simulink model "HuskyFullSim_TorqueControl"  (R2025a)
settings: Solver=VariableStepAuto  StartTime=0.0  StopTime=1  RelTol=1e-5  AbsTol=1e-5  EnableMultiTasking=on
undefined symbols (not defined in the file): X, Y, Z
libraries: sm_lib x83, nesl_utility x81
(part 1 of 4)
settings Model: Creator=Prath  LastModifiedBy=Prath
settings SolverCC: AutoScaleAbsTol=off  AlgebraicLoopSolver=TrustRegion  MaxZcPerStep=1.0
settings DataIOCC: LimitDataPoints=on  MaxDataPoints=10000
settings OptimizationCC: ReuseModelBlockBuffer=off  LifeSpan=inf
settings DebuggingCC: UnconnectedInputMsg=warning  UnconnectedOutputMsg=warning  UnconnectedLineMsg=warning  AllowSymbolicDim=off  SubsystemReferenceDiagnosticForUnitTest=warning  SFUnexpectedBacktrackingDiag=warning  SFNoUnconditionalDefaultTransitionDiag=warning  SFExecutionAtInitializationDiag=none  ArithmeticOperatorsInVariantConditions=warning
settings ModelReferenceCC: EnableRefExpFcnMdlSchedulingChecks=on
settings SFSimCC: SimUseLocalCustomCode=off  CustomCodeUndefinedFunction=UseInterfaceOnly
settings RTWCC: RTWUseLocalCustomCode=off  GPUComputeCapability=3.5  DLArmComputeVersion=19.05
settings CodeAppCC: StateflowObjectComments=on
settings GRTTargetCC: TargetLangStandard=C89/C90 (ANSI)
settings ConfigComp: CovMetricSettings=dw  CovSaveCumulativeToWorkspaceVar=on  CovSaveSingleToWorkspaceVar=on  CovExternalEMLEnable=off  CovSFcnEnable=off
settings SimscapeCC: SimscapeLogType=all  SimscapeLogSimulationStatistics=on  SimscapeLogDataHistory=10000.0
settings ExplorerConfigSet: InternalSimMechanicsExplorerSettings="<ExplorerConfiguration><canonicalview>default</canonicalview><TilePanel><TileInfo><Tiles Columns=\"1\" Count=\"1\" Height=\"824\" Rows=\"1\" Width=\"1703\"><Row Weight=\"1\"/><Column Weight=\"1\"/><Tile Height=\"1\" Width=\"1\" X=\"0\" Y=\"0\"/></Tiles></TileInfo><SceneInfo><SceneViewer><IsThisViewStd><IsStandardView>off</IsStandardView><StandardViewName>Front</StandardViewName></IsThisViewStd><BGColor><R>1</R><G>1</G><B>1</B><A>1</A></BGColor><Camera><DoPerspective>off</DoPerspective><Position><X>-0.84082597181311081</X><Y>0.97301356742484102</Y><Z>-0.37165255861931379</Z></Position><Center><X>0.16436719658721111</X><Y>-0.14249902054546354</Y><Z>-0.28624750343827171</Z></Center><Up><X>0.59851844460548564</X><Y>0.58151391770421146</Y><Z>0.55101473209282714</Z></Up><XLim>0.64254437732877001</XLim><YLim>0.64254437732877001</YLim><ViewLimDist>0.01</ViewLimDist></Camera></SceneViewer></SceneInfo></TilePanel><MechEditorPanel><GfxPanelCameraMap/><Cameras/><VideoCreator><IncludeTiles>All</IncludeTiles><IncludeTime>on</IncludeTime><IncludeWorldFrame>off</IncludeWorldFrame><PlaybackSpeedRatio>1</PlaybackSpeedRatio><FrameRate>60</FrameRate><FrameSize>auto</FrameSize><VideoFormat>MPEG4</VideoFormat></VideoCreator></MechEditorPanel><PlaybackSettings><PlaybackSpeedFactor>1</PlaybackSpeedFactor></PlaybackSettings></ExplorerConfiguration>"

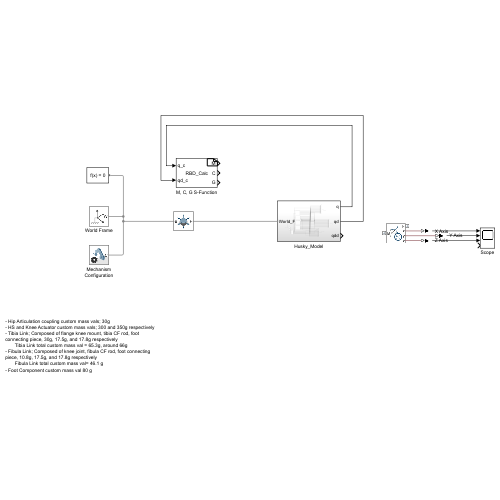
[thumbnail: Simulink's stored preview of the top-level diagram]
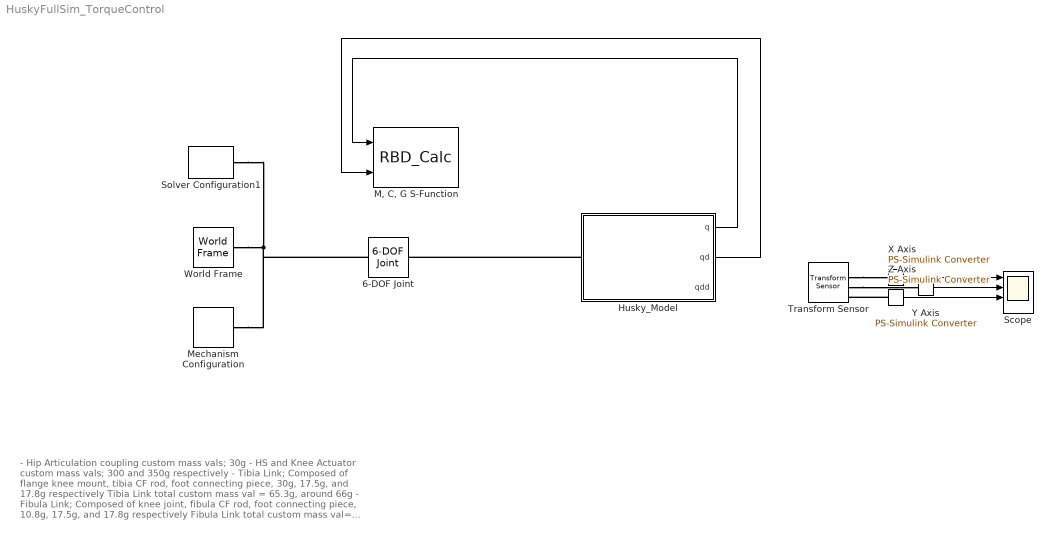
== system HuskyFullSim_TorqueControl ==
  note: - Hip Articulation coupling custom mass vals; 30g
      | - HS and Knee Actuator custom mass vals; 300 and 350g respectively
      | - Tibia Link; Composed of flange knee mount, tibia CF rod, foot connecting piece, 30g, 17.5g, and 17.8g respectively
      | Tibia Link total custom mass val = 65.3g, around 66g
      | - Fibula Link; Composed of knee joint, fibula CF rod, foot connecting piece, 10.8g, 17.5g, and 17.8g respectively
      | Fibula Link total custom mass val= 46.1 g
      | - Foot Component custom mass val 80 g
  6-DOF Joint : sm_lib/Joints/6-DOF Joint  JointMode=Normal  CompositeWrenchDir=FollowerOnBase  CompositeWrenchFrame=BaseFrame  SenseConstraintForce=off  SenseConstraintTorque=off  SenseTotalForce=off  SenseTotalTorque=off  PxPositionTargetSpecify=off  PxPositionTargetPriority=High  PxPositionTargetValue=0  PxPositionTargetValueUnits=m  PxVelocityTargetSpecify=off  PxVelocityTargetPriority=High  PxVelocityTargetValue=0  PxVelocityTargetValueUnits=m/s  PxEquilibriumPosition=0  PxEquilibriumPositionUnits=m  PxSpringStiffness=0  PxSpringStiffnessUnits=N/m  PxDampingCoefficient=0  PxDampingCoefficientUnits=N/(m/s)  PxLowerLimitSpecify=off  PxLowerLimitBound=-1  PxLowerLimitBoundUnits=m  PxLowerLimitStiffness=1e6  PxLowerLimitStiffnessUnits=N/m  PxLowerLimitDamping=1e3  PxLowerLimitDampingUnits=N/(m/s)  PxLowerLimitTransitionRegionWidth=1e-4  PxLowerLimitTransitionRegionWidthUnits=m  PxUpperLimitSpecify=off  PxUpperLimitBound=1  PxUpperLimitBoundUnits=m  PxUpperLimitStiffness=1e6  PxUpperLimitStiffnessUnits=N/m  PxUpperLimitDamping=1e3  PxUpperLimitDampingUnits=N/(m/s)  PxUpperLimitTransitionRegionWidth=1e-4  PxUpperLimitTransitionRegionWidthUnits=m  PxTorqueActuationMode=NoTorque  PxMotionActuationMode=ComputedMotion  PxSensePosition=off  PxSenseVelocity=off  PxSenseAcceleration=off  PxSenseTorqueForce=off  PxSenseLowerLimitTorqueForce=off  PxSenseUpperLimitTorqueForce=off  PyPositionTargetSpecify=off  PyPositionTargetPriority=High  PyPositionTargetValue=0  PyPositionTargetValueUnits=m  PyVelocityTargetSpecify=off  PyVelocityTargetPriority=High  PyVelocityTargetValue=0  PyVelocityTargetValueUnits=m/s  PyEquilibriumPosition=0  PyEquilibriumPositionUnits=m  PySpringStiffness=0  PySpringStiffnessUnits=N/m  PyDampingCoefficient=0  PyDampingCoefficientUnits=N/(m/s)  PyLowerLimitSpecify=off  PyLowerLimitBound=-1  PyLowerLimitBoundUnits=m  PyLowerLimitStiffness=1e6  PyLowerLimitStiffnessUnits=N/m  PyLowerLimitDamping=1e3  PyLowerLimitDampingUnits=N/(m/s)  PyLowerLimitTransitionRegionWidth=1e-4  PyLowerLimitTransitionRegionWidthUnits=m  PyUpperLimitSpecify=off  PyUpperLimitBound=1  PyUpperLimitBoundUnits=m  PyUpperLimitStiffness=1e6  PyUpperLimitStiffnessUnits=N/m  PyUpperLimitDamping=1e3  PyUpperLimitDampingUnits=N/(m/s)  PyUpperLimitTransitionRegionWidth=1e-4  PyUpperLimitTransitionRegionWidthUnits=m  PyTorqueActuationMode=NoTorque  PyMotionActuationMode=ComputedMotion  PySensePosition=off  PySenseVelocity=off  PySenseAcceleration=off  PySenseTorqueForce=off  PySenseLowerLimitTorqueForce=off  PySenseUpperLimitTorqueForce=off  PzPositionTargetSpecify=off  PzPositionTargetPriority=High  PzPositionTargetValue=0  PzPositionTargetValueUnits=m  PzVelocityTargetSpecify=off  PzVelocityTargetPriority=High  PzVelocityTargetValue=0  PzVelocityTargetValueUnits=m/s  PzEquilibriumPosition=0  PzEquilibriumPositionUnits=m  PzSpringStiffness=0  PzSpringStiffnessUnits=N/m  PzDampingCoefficient=0  PzDampingCoefficientUnits=N/(m/s)  PzLowerLimitSpecify=off  PzLowerLimitBound=-1  PzLowerLimitBoundUnits=m  PzLowerLimitStiffness=1e6  PzLowerLimitStiffnessUnits=N/m  PzLowerLimitDamping=1e3  PzLowerLimitDampingUnits=N/(m/s)  PzLowerLimitTransitionRegionWidth=1e-4  PzLowerLimitTransitionRegionWidthUnits=m  PzUpperLimitSpecify=off  PzUpperLimitBound=1  PzUpperLimitBoundUnits=m  PzUpperLimitStiffness=1e6  PzUpperLimitStiffnessUnits=N/m  PzUpperLimitDamping=1e3  PzUpperLimitDampingUnits=N/(m/s)  PzUpperLimitTransitionRegionWidth=1e-4  PzUpperLimitTransitionRegionWidthUnits=m  PzTorqueActuationMode=NoTorque  PzMotionActuationMode=ComputedMotion  PzSensePosition=off  PzSenseVelocity=off  PzSenseAcceleration=off  PzSenseTorqueForce=off  PzSenseLowerLimitTorqueForce=off  PzSenseUpperLimitTorqueForce=off  SphPositionTargetSpecify=off  SphPositionTargetPriority=High  SphPositionTargetRotationMethod=None  SphPositionTargetFollAlignAxisA=+X  SphPositionTargetBaseAlignAxisA=+Y  SphPositionTargetFollAlignAxisB=+Y  SphPositionTargetBaseAlignAxisB=+Z  SphPositionTargetRotationStandardAxis=+Z  SphPositionTargetRotationAngle=0  SphPositionTargetRotationAngleUnits=deg  SphPositionTargetRotationArbitraryAxis=[0 0 1]  SphPositionTargetRotationSequenceAxes=FollowerAxes  SphPositionTargetRotationSequence=XYX  SphPositionTargetRotationSequenceAngles=[0 0 0]  SphPositionTargetRotationSequenceAnglesUnits=deg  SphPositionTargetRotationMatrix=[1 0 0;0 1 0;0 0 1]  SphPositionTargetQuaternion=[1 0 0 0]  SphVelocityTargetSpecify=off  SphVelocityTargetPriority=High  SphVelocityTargetValue=[0 0 0]  SphVelocityTargetValueUnits=deg/s  SphVelocityTargetInFollowerFrame=on  SphEqPosRotationMethod=None  SphEqPosFollAlignAxisA=+X  SphEqPosBaseAlignAxisA=+Y  SphEqPosFollAlignAxisB=+Y  SphEqPosBaseAlignAxisB=+Z  SphEqPosRotationStandardAxis=+Z  SphEqPosRotationAngle=0  SphEqPosRotationAngleUnits=deg  SphEqPosRotationArbitraryAxis=[0 0 1]  SphEqPosRotationSequenceAxes=FollowerAxes  SphEqPosRotationSequence=XYX  SphEqPosRotationSequenceAngles=[0 0 0]  SphEqPosRotationSequenceAnglesUnits=deg  SphEqPosRotationMatrix=[1 0 0;0 1 0;0 0 1]  SphEqPosQuaternion=[1 0 0 0]  SphSpringStiffness=0  SphSpringStiffnessUnits=N*m/deg  SphDampingCoefficient=0  SphDampingCoefficientUnits=N*m/(deg/s)  SphLowerLimitSpecify=off  SphLowerLimitBound=15  SphLowerLimitBoundUnits=deg  SphLowerLimitStiffness=1e4  SphLowerLimitStiffnessUnits=N*m/deg  SphLowerLimitDamping=10  SphLowerLimitDampingUnits=N*m/(deg/s)  SphLowerLimitTransitionRegionWidth=0.1  SphLowerLimitTransitionRegionWidthUnits=deg  SphUpperLimitSpecify=off  SphUpperLimitBound=45  SphUpperLimitBoundUnits=deg  SphUpperLimitStiffness=1e4  SphUpperLimitStiffnessUnits=N*m/deg  SphUpperLimitDamping=10  SphUpperLimitDampingUnits=N*m/(deg/s)  SphUpperLimitTransitionRegionWidth=0.1  SphUpperLimitTransitionRegionWidthUnits=deg  SphTorqueActuationMode=NoTorque  SphActuateTorqueX=off  SphActuateTorqueY=off  SphActuateTorqueZ=off  SphActuateTorque=off  SphActuationFrame=BaseFrame  SphSensePosition=off  SphSenseVelocityX=off  SphSenseVelocityY=off  SphSenseVelocityZ=off  SphSenseVelocity=off  SphSenseAccelerationX=off  SphSenseAccelerationY=off  SphSenseAccelerationZ=off  SphSenseAcceleration=off  SphSenseLowerLimitTorqueMag=off  SphSenseUpperLimitTorqueMag=off  SphSensingFrame=BaseFrame
  Husky_Model : Subsystem
  "M, C, G S-Function" : S-Function  FunctionName=RBD_Calc  SFunctionDeploymentMode=off  EnableBusSupport=off  mask(S-Function Builder){}
      mask help: Simulink:masks:SFunctionBuilder_MD
      mask init:
      | val = [[.9  0.75 0.75 1 1 .9 .9 1]',[1 1 0.75 0.75 .9 .9 1 .9]'];try , sys = get_param(gcb,'SfunBuilderFcnName');if isempty(sys), sys = get_param(gcb,'FunctionName'); end,catch, sys = get_param(gcb,'FunctionName'); end
      settings: CopyFcn=set_param(gcbh,'LinkStatus','none')  OpenFcn=sfunctionwizard(gcbh)
      mask Display: plot(val(:,1),val(:,2)),disp(sys),port_label('input',1,'q_c'),port_label('input',2,'qd_c'),port_label('output',1,'M'),port_label('output',2,'C'),port_label('output',3,'G')
  Mechanism Configuration : sm_lib/Utilities/Mechanism Configuration  UniformGravity=Constant  GravityVector=[0 0 -9.80665]  GravityVectorUnits=m/s^2  LinearizationDelta=0.001  JointModeTransitionNonlinearIterations=2
  Scope : Scope  NumInputPorts=4
      settings: ActiveDisplayYMinimum=-0.0061861791306105857  ActiveDisplayYMaximum=0.0040663833622028378
  Solver Configuration1 : nesl_utility/Solver Configuration  PhysicalDomain=network_engine_domain  SubClassName=solver  LeftPortType=input  RightPortType=generic  Tones=[]  Harmonics=[]  SimulateNoise=off  Profile=off  UseLocalSampling=off  EnableSwitchedLinearOptims=on  FrequencyDomain=off  UseCCode=off  RelTol=0.001  AbsTol=0.001  MinStep=1e-09  ToWorkspace=off  RevertToSquareIcSolve=off  NumHomotopyIterations=100  PhasorMode=off  PhasorModeNumHarmonics=1  ConsistencySolver=NEWTON_XTOL_AFTER_FTOL  IndexReductionMethod=DerivativeReplacement  DoDC=off  ResidualTolerance=1e-09  ConsistencyTolSource=GLOBAL  ConsistencyAbsTol=0.001  ConsistencyRelTol=0.001  ConsistencyTolFactor=0.001  UseLocalSolver=on  LocalSolverChoice=NE_BACKWARD_EULER_ADVANCER  ResolveIndetEquations=on  FunctionEvalNumThread=1  LocalSolverSampleTime=0.001  DoFixedCost=off  MaxNonlinIter=3  MaxModeIter=2  ComputeImpulses=off  ImpulseIterations=2  LinearAlgebra=auto  LinearAlgebraNumThread=0  EquationFormulation=NE_FREQUENCY_TIME_EF  DelaysMemoryBudget=1024  AutomaticFiltering=on  FilteringTimeConstant=0.001  PartitionStorageMethod=AS_NEEDED  PartitionMemoryBudget=1024  PartitionMethod=ROBUST  MultibodyUseLocalSolver=on  MultibodyLocalSolverChoice=ODE3  MultibodyLocalSolverSampleTime=0.001
  Transform Sensor : sm_lib/Frames and Transforms/Transform Sensor  MeasurementFrame=World  RotationSequence=XYX  SenseAngle=off  SenseAxis=off  SenseQ=off  SenseR=off  SenseRotationSequence=off  SenseOmegaX=off  SenseOmegaY=off  SenseOmegaZ=off  SenseOmega=off  SenseQDot=off  SenseRDot=off  SenseRotationSequenceDot=off  SenseAlphaX=off  SenseAlphaY=off  SenseAlphaZ=off  SenseAlpha=off  SenseQDDot=off  SenseRDDot=off  SenseX=on  SenseY=on  SenseZ=on  SenseXYZ=off  SenseRad=off  SenseAzim=off  SenseDist=off  SenseInc=off  SenseXDot=off  SenseYDot=off  SenseZDot=off  SenseXYZDot=off  SenseRadDot=off  SenseAzimDot=off  SenseDistDot=off  SenseIncDot=off  SenseXDDot=off  SenseYDDot=off  SenseZDDot=off  SenseXYZDDot=off  SenseRadDDot=off  SenseAzimDDot=off  SenseDistDDot=off  SenseIncDDot=off
  World Frame : sm_lib/Frames and Transforms/World Frame
  X Axis : nesl_utility/PS-Simulink Converter  PhysicalDomain=network_engine_domain  SubClassName=ps_output  LeftPortType=input  RightPortType=output  PseudoPeriodic=off  Frequencies=[]  VectorFormat=inherit  Unit=inherit  AffineConversion=off
  Y Axis : nesl_utility/PS-Simulink Converter  PhysicalDomain=network_engine_domain  SubClassName=ps_output  LeftPortType=input  RightPortType=output  PseudoPeriodic=off  Frequencies=[]  VectorFormat=inherit  Unit=inherit  AffineConversion=off
  Z Axis : nesl_utility/PS-Simulink Converter  PhysicalDomain=network_engine_domain  SubClassName=ps_output  LeftPortType=input  RightPortType=output  PseudoPeriodic=off  Frequencies=[]  VectorFormat=inherit  Unit=inherit  AffineConversion=off
  wires:
  X Axis/1 -> Scope/1
  Y Axis/1 -> Scope/2
  Z Axis/1 -> Scope/3
  Husky_Model/1(q) -> "M, C, G S-Function"/1
  Husky_Model/2(qd) -> "M, C, G S-Function"/2
  connections:
  World Frame/RConn1 -- Solver Configuration1/RConn1 -- 6-DOF Joint/LConn1 -- Mechanism Configuration/RConn1
  Transform Sensor/RConn2 -- X Axis/LConn1
  Transform Sensor/RConn3 -- Y Axis/LConn1
  Z Axis/LConn1 -- Transform Sensor/RConn4
  Husky_Model/LConn1 -- 6-DOF Joint/RConn1

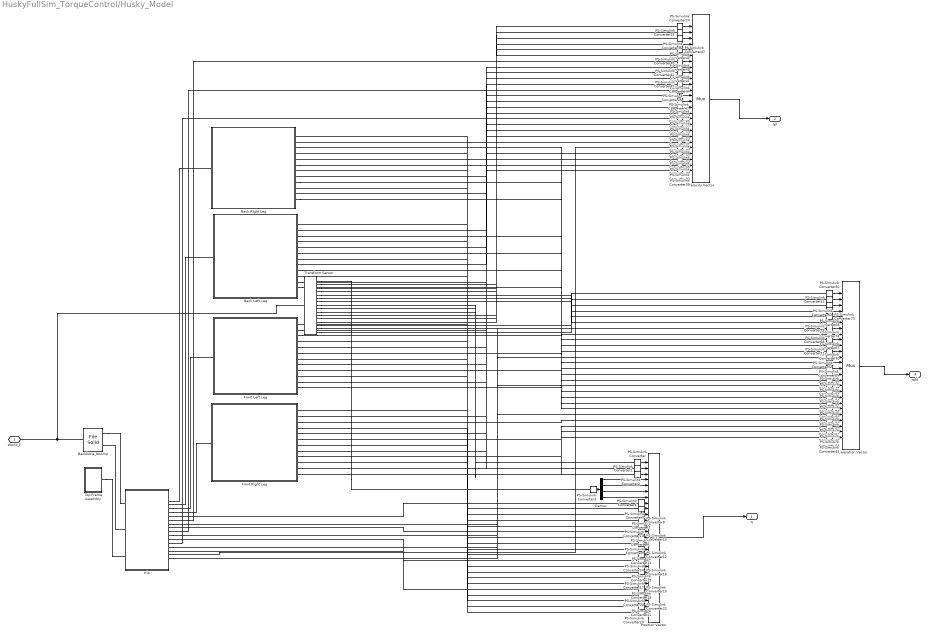
== system HuskyFullSim_TorqueControl/Husky_Model ==
  Acceleration Vector : Mux  Inputs=26
  Back Left Leg : Subsystem
  Back Right Leg : Subsystem
  Backbone_NoAmp : sm_lib/Body Elements/File Solid  ExtGeomFileName=C:\Users\Prath\OneDrive\Documents\MATLAB\Backbone_Assy_NoAmp.STEP  UnitType=FromFile  ExtGeomFileUnits=m  StepReaderType=HEX  ExportConvexHullGeometry=off  InertiaType=CalculateFromGeometry  BasedOnType=Mass  Density=1000  DensityUnits=kg/m^3  Mass=1.5  MassUnits=kg  CenterOfMass=[0 0 0]  CenterOfMassUnits=m  MomentsOfInertia=[1 1 1]  MomentsOfInertiaUnits=kg*m^2  ProductsOfInertia=[0 0 0]  ProductsOfInertiaUnits=kg*m^2  GraphicType=FromGeometry  MarkerShape=Sphere  MarkerSize=10  GraphicVisPropType=SimpleVisualProperties  GraphicDiffuseColor=[0.5 0.5 0.5]  GraphicOpacity=1  GraphicSpecularColor=[0.5 0.5 0.5 1.0]  GraphicAmbientColor=[0.15 0.15 0.15 1.0]  GraphicEmissiveColor=[0.0 0.0 0.0 1.0]  GraphicShininess=75  DoExposeReferenceFrame=on  SerializedFrames=<Frames><Frame><Id>Frame1</Id><Value><Name>F1</Name><Origin><Source>GeometricFeature</Source><FeatureName>planar surface 366</FeatureName></Origin><PrimaryAxis><DefinedDirection>+Z</DefinedDirection><Source>ReferenceFrame</Source><SourceDirection>+Z</SourceDirection><FeatureName></FeatureName></PrimaryAxis><SecondaryAxis><DefinedDirection>+X</DefinedDirection><Source>ReferenceFrame</Source><SourceDirection>+X</SourceDirection><FeatureName></FeatureName></SecondaryAxis></Value></Frame><Frame><Id>Frame2</Id><Value><Name>F2</Name><Origin><Source>GeometricFeature</Source><FeatureName>planar surface 599</FeatureName></Origin><PrimaryAxis><DefinedDirection>+Z</DefinedDirection><Source>ReferenceFrame</Source><SourceDirection>+Z</SourceDirection><FeatureName></FeatureName></PrimaryAxis><SecondaryAxis><DefinedDirection>+X</DefinedDirection><Source>ReferenceFrame</Source><SourceDirection>+X</SourceDirection><FeatureName></FeatureName></SecondaryAxis></Value></Frame></Frames>
  Demux : Demux
  Front Left Leg : Subsystem
  Front Right Leg : Subsystem
  Hip : Subsystem
  PS-Simulink Converter{,1..75} (76 alike) : nesl_utility/PS-Simulink Converter  PhysicalDomain=network_engine_domain  SubClassName=ps_output  LeftPortType=input  RightPortType=output  PseudoPeriodic=off  Frequencies=[]  VectorFormat=inherit  Unit=inherit  AffineConversion=off
  Position Vector : Mux  Inputs=27
  Top Frame Assembly : Subsystem
  Transform Sensor : sm_lib/Frames and Transforms/Transform Sensor  MeasurementFrame=World  RotationSequence=XYX  SenseAngle=off  SenseAxis=off  SenseQ=on  SenseR=off  SenseRotationSequence=off  SenseOmegaX=on  SenseOmegaY=on  SenseOmegaZ=on  SenseOmega=off  SenseQDot=off  SenseRDot=off  SenseRotationSequenceDot=off  SenseAlphaX=on  SenseAlphaY=on  SenseAlphaZ=on  SenseAlpha=off  SenseQDDot=off  SenseRDDot=off  SenseX=on  SenseY=on  SenseZ=on  SenseXYZ=off  SenseRad=off  SenseAzim=off  SenseDist=off  SenseInc=off  SenseXDot=on  SenseYDot=on  SenseZDot=on  SenseXYZDot=off  SenseRadDot=off  SenseAzimDot=off  SenseDistDot=off  SenseIncDot=off  SenseXDDot=on  SenseYDDot=on  SenseZDDot=on  SenseXYZDDot=off  SenseRadDDot=off  SenseAzimDDot=off  SenseDistDDot=off  SenseIncDDot=off
  Velocity Vector : Mux  Inputs=26
  World_F : PMIOPort  Side=Left
  q : Outport
  qd : Outport  Port=2
  qdd : Outport  Port=3
  wires:
  PS-Simulink Converter/1 -> Position Vector/1
  PS-Simulink Converter1/1 -> Position Vector/2
  PS-Simulink Converter2/1 -> Position Vector/3
  PS-Simulink Converter3/1 -> Demux/1
  Demux/1 -> Position Vector/4
  Demux/2 -> Position Vector/5
  Demux/3 -> Position Vector/6
  Demux/4 -> Position Vector/7
  PS-Simulink Converter6/1 -> Position Vector/13
  PS-Simulink Converter4/1 -> Position Vector/8
  PS-Simulink Converter5/1 -> Position Vector/9
  PS-Simulink Converter7/1 -> Position Vector/10
  PS-Simulink Converter8/1 -> Position Vector/11
  PS-Simulink Converter13/1 -> Position Vector/14
  PS-Simulink Converter12/1 -> Position Vector/17
  PS-Simulink Converter11/1 -> Position Vector/16
  PS-Simulink Converter9/1 -> Position Vector/15
  PS-Simulink Converter10/1 -> Position Vector/12
  PS-Simulink Converter14/1 -> Position Vector/18
  PS-Simulink Converter15/1 -> Position Vector/19
  PS-Simulink Converter16/1 -> Position Vector/20
  PS-Simulink Converter17/1 -> Position Vector/21
  PS-Simulink Converter18/1 -> Position Vector/22
  PS-Simulink Converter19/1 -> Position Vector/23
  PS-Simulink Converter20/1 -> Position Vector/24
  PS-Simulink Converter22/1 -> Position Vector/26
  PS-Simulink Converter21/1 -> Position Vector/25
  PS-Simulink Converter23/1 -> Position Vector/27
  PS-Simulink Converter25/1 -> Velocity Vector/2
  PS-Simulink Converter32/1 -> Velocity Vector/20
  PS-Simulink Converter28/1 -> Velocity Vector/17
  PS-Simulink Converter24/1 -> Velocity Vector/1
  PS-Simulink Converter46/1 -> Velocity Vector/15
  PS-Simulink Converter26/1 -> Velocity Vector/12
  PS-Simulink Converter42/1 -> Velocity Vector/9
  PS-Simulink Converter44/1 -> Velocity Vector/10
  PS-Simulink Converter35/1 -> Velocity Vector/23
  PS-Simulink Converter34/1 -> Velocity Vector/22
  PS-Simulink Converter39/1 -> Velocity Vector/26
  PS-Simulink Converter36/1 -> Velocity Vector/3
  PS-Simulink Converter29/1 -> Velocity Vector/14
  PS-Simulink Converter41/1 -> Velocity Vector/8
  PS-Simulink Converter43/1 -> Velocity Vector/13
  PS-Simulink Converter33/1 -> Velocity Vector/21
  PS-Simulink Converter37/1 -> Velocity Vector/24
  PS-Simulink Converter27/1 -> Velocity Vector/16
  PS-Simulink Converter30/1 -> Velocity Vector/18
  PS-Simulink Converter31/1 -> Velocity Vector/19
  PS-Simulink Converter45/1 -> Velocity Vector/11
  PS-Simulink Converter38/1 -> Velocity Vector/25
  PS-Simulink Converter40/1 -> Velocity Vector/4
  PS-Simulink Converter47/1 -> Velocity Vector/5
  PS-Simulink Converter48/1 -> Velocity Vector/6
  PS-Simulink Converter49/1 -> Velocity Vector/7
  PS-Simulink Converter73/1 -> Acceleration Vector/5
  PS-Simulink Converter64/1 -> Acceleration Vector/25
  PS-Simulink Converter69/1 -> Acceleration Vector/13
  PS-Simulink Converter53/1 -> Acceleration Vector/16
  PS-Simulink Converter67/1 -> Acceleration Vector/8
  PS-Simulink Converter59/1 -> Acceleration Vector/21
  PS-Simulink Converter55/1 -> Acceleration Vector/14
  PS-Simulink Converter71/1 -> Acceleration Vector/11
  PS-Simulink Converter57/1 -> Acceleration Vector/19
  PS-Simulink Converter62/1 -> Acceleration Vector/3
  PS-Simulink Converter56/1 -> Acceleration Vector/18
  PS-Simulink Converter68/1 -> Acceleration Vector/9
  PS-Simulink Converter61/1 -> Acceleration Vector/23
  PS-Simulink Converter50/1 -> Acceleration Vector/1
  PS-Simulink Converter63/1 -> Acceleration Vector/24
  PS-Simulink Converter58/1 -> Acceleration Vector/20
  PS-Simulink Converter72/1 -> Acceleration Vector/15
  PS-Simulink Converter52/1 -> Acceleration Vector/12
  PS-Simulink Converter54/1 -> Acceleration Vector/17
  PS-Simulink Converter60/1 -> Acceleration Vector/22
  PS-Simulink Converter51/1 -> Acceleration Vector/2
  PS-Simulink Converter65/1 -> Acceleration Vector/26
  PS-Simulink Converter74/1 -> Acceleration Vector/6
  PS-Simulink Converter75/1 -> Acceleration Vector/7
  PS-Simulink Converter66/1 -> Acceleration Vector/4
  PS-Simulink Converter70/1 -> Acceleration Vector/10
  Position Vector/1 -> q/1
  Velocity Vector/1 -> qd/1
  Acceleration Vector/1 -> qdd/1
  connections:
  Back Left Leg/LConn1 -- Hip/RConn2
  Backbone_NoAmp/RConn1 -- Transform Sensor/LConn1 -- World_F/RConn1
  Top Frame Assembly/RConn1 -- Hip/LConn3
  Hip/LConn2 -- Backbone_NoAmp/LConn2
  Hip/RConn3 -- Front Left Leg/LConn1
  Back Right Leg/LConn1 -- Hip/RConn1
  Hip/RConn4 -- Front Right Leg/LConn1
  Backbone_NoAmp/LConn1 -- Hip/LConn1
  Transform Sensor/RConn9 -- PS-Simulink Converter/LConn1
  Transform Sensor/RConn10 -- PS-Simulink Converter1/LConn1
  Transform Sensor/RConn11 -- PS-Simulink Converter2/LConn1
  Transform Sensor/RConn2 -- PS-Simulink Converter3/LConn1
  PS-Simulink Converter5/LConn1 -- Back Left Leg/RConn1
  PS-Simulink Converter4/LConn1 -- Hip/RConn5
  PS-Simulink Converter7/LConn1 -- Back Left Leg/RConn4
  PS-Simulink Converter8/LConn1 -- Back Left Leg/RConn7
  PS-Simulink Converter10/LConn1 -- Back Left Leg/RConn10
  PS-Simulink Converter6/LConn1 -- Hip/RConn8
  PS-Simulink Converter13/LConn1 -- Back Right Leg/RConn1
  PS-Simulink Converter9/LConn1 -- Back Right Leg/RConn4
  PS-Simulink Converter11/LConn1 -- Back Right Leg/RConn10
  PS-Simulink Converter12/LConn1 -- Back Right Leg/RConn7
  PS-Simulink Converter14/LConn1 -- Hip/RConn11
  PS-Simulink Converter15/LConn1 -- Front Left Leg/RConn1
  PS-Simulink Converter16/LConn1 -- Front Left Leg/RConn4
  PS-Simulink Converter17/LConn1 -- Front Left Leg/RConn7
  PS-Simulink Converter18/LConn1 -- Front Left Leg/RConn10
  PS-Simulink Converter19/LConn1 -- Hip/RConn14
  PS-Simulink Converter20/LConn1 -- Front Right Leg/RConn1
  Front Right Leg/RConn4 -- PS-Simulink Converter21/LConn1
  PS-Simulink Converter22/LConn1 -- Front Right Leg/RConn7
  PS-Simulink Converter23/LConn1 -- Front Right Leg/RConn10
  Transform Sensor/RConn12 -- PS-Simulink Converter24/LConn1
  Transform Sensor/RConn13 -- PS-Simulink Converter25/LConn1
  Transform Sensor/RConn14 -- PS-Simulink Converter36/LConn1
  Transform Sensor/RConn3 -- PS-Simulink Converter40/LConn1
  Transform Sensor/RConn4 -- PS-Simulink Converter47/LConn1
  Transform Sensor/RConn5 -- PS-Simulink Converter48/LConn1
  PS-Simulink Converter49/LConn1 -- Hip/RConn6
  PS-Simulink Converter41/LConn1 -- Back Left Leg/RConn2
  PS-Simulink Converter42/LConn1 -- Back Left Leg/RConn5
  PS-Simulink Converter44/LConn1 -- Back Left Leg/RConn8
  Back Left Leg/RConn11 -- PS-Simulink Converter45/LConn1
  PS-Simulink Converter26/LConn1 -- Hip/RConn9
  PS-Simulink Converter43/LConn1 -- Back Right Leg/RConn2
  PS-Simulink Converter29/LConn1 -- Back Right Leg/RConn5
  PS-Simulink Converter46/LConn1 -- Back Right Leg/RConn11
  PS-Simulink Converter27/LConn1 -- Back Right Leg/RConn8
  PS-Simulink Converter28/LConn1 -- Hip/RConn12
  Front Left Leg/RConn2 -- PS-Simulink Converter30/LConn1
  Front Left Leg/RConn5 -- PS-Simulink Converter31/LConn1
  Front Left Leg/RConn8 -- PS-Simulink Converter32/LConn1
  Front Left Leg/RConn11 -- PS-Simulink Converter33/LConn1
  PS-Simulink Converter34/LConn1 -- Hip/RConn15
  Front Right Leg/RConn2 -- PS-Simulink Converter35/LConn1
  Front Right Leg/RConn5 -- PS-Simulink Converter37/LConn1
  Front Right Leg/RConn8 -- PS-Simulink Converter38/LConn1
  Front Right Leg/RConn11 -- PS-Simulink Converter39/LConn1
  Transform Sensor/RConn15 -- PS-Simulink Converter50/LConn1
  Transform Sensor/RConn17 -- PS-Simulink Converter62/LConn1
  Transform Sensor/RConn16 -- PS-Simulink Converter51/LConn1
  Transform Sensor/RConn7 -- PS-Simulink Converter73/LConn1
  Transform Sensor/RConn6 -- PS-Simulink Converter66/LConn1
  Transform Sensor/RConn8 -- PS-Simulink Converter74/LConn1
  Hip/RConn7 -- PS-Simulink Converter75/LConn1
  Hip/RConn10 -- PS-Simulink Converter52/LConn1
  Hip/RConn13 -- PS-Simulink Converter54/LConn1
  Hip/RConn16 -- PS-Simulink Converter60/LConn1
  Back Left Leg/RConn3 -- PS-Simulink Converter67/LConn1
  Back Left Leg/RConn6 -- PS-Simulink Converter68/LConn1
  Back Left Leg/RConn9 -- PS-Simulink Converter70/LConn1
  Back Left Leg/RConn12 -- PS-Simulink Converter71/LConn1
  Back Right Leg/RConn3 -- PS-Simulink Converter69/LConn1
  Back Right Leg/RConn6 -- PS-Simulink Converter55/LConn1
  Back Right Leg/RConn12 -- PS-Simulink Converter72/LConn1
  Back Right Leg/RConn9 -- PS-Simulink Converter53/LConn1
  Front Left Leg/RConn3 -- PS-Simulink Converter56/LConn1
  Front Left Leg/RConn6 -- PS-Simulink Converter57/LConn1
  Front Left Leg/RConn9 -- PS-Simulink Converter58/LConn1
  Front Left Leg/RConn12 -- PS-Simulink Converter59/LConn1
  Front Right Leg/RConn3 -- PS-Simulink Converter61/LConn1
  Front Right Leg/RConn6 -- PS-Simulink Converter63/LConn1
  Front Right Leg/RConn9 -- PS-Simulink Converter64/LConn1
  Front Right Leg/RConn12 -- PS-Simulink Converter65/LConn1
